simulink model "Linearisierung3_RoboKomplettmodell_Sim"  (R2017a)
settings: Solver=VariableStepAuto  StartTime=0.0  StopTime=50  RelTol=1e-3
values from neighbouring files (symbols this model uses):
  c = 1    [Linearisierung3_Robo.m]
  g = 9.81    [Linearisierung3_Robo.m]
  K = 300    [Linearisierung3_Robo.m]
  l = 1    [Linearisierung3_Robo.m]
  m = 7    [Linearisierung3_Robo.m]
  T = 0.1    [Linearisierung3_Robo.m]
settings Model: Creator=jonas  LastModifiedBy=Jonas

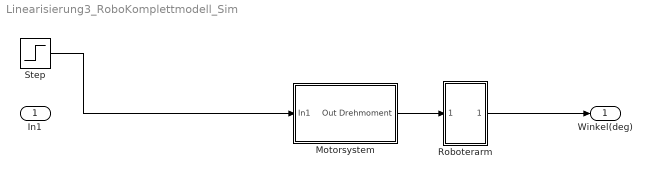
== system Linearisierung3_RoboKomplettmodell_Sim ==
  In1 : Inport
  Motorsystem : Subsystem
  Roboterarm : Subsystem
  Step : Step  After=0.1471  SampleTime=0
  Winkel(deg) : Outport
  wires:
  Motorsystem/1(Out Drehmoment) -> Roboterarm/1(In1)
  Roboterarm/1(Out1) -> Winkel(deg)/1
  Step/1 -> Motorsystem/1(In1)

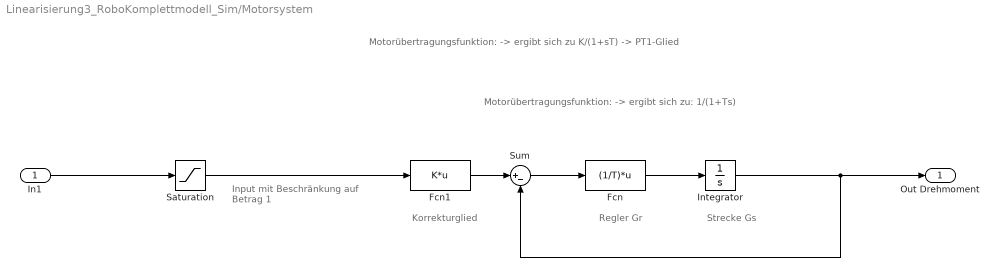
== system Linearisierung3_RoboKomplettmodell_Sim/Motorsystem ==
  note: Motorübertragungsfunktion:
      |  -> ergibt sich zu K/(1+sT)
      |  -> PT1-Glied
  note: Motorübertragungsfunktion:
      |  -> ergibt sich zu: 1/(1+Ts)
  note: Korrekturglied
  note: Input
      | mit Beschränkung
      | auf Betrag 1
  note: Regler Gr
  note: Strecke Gs
  In1 : Inport
  Fcn : Fcn  Expr=(1/T)*u
  Fcn1 : Fcn  Expr=K*u
  Integrator : Integrator
  Saturation : Saturate  UpperLimit=1  LowerLimit=-1
  Sum : Sum  Inputs=|+-
  Out Drehmoment : Outport
  wires:
  Fcn1/1 -> Sum/1
  Fcn/1 -> Integrator/1
  Integrator/1 -> Out Drehmoment/1, Sum/2
  Saturation/1 -> Fcn1/1
  Sum/1 -> Fcn/1
  In1/1 -> Saturation/1

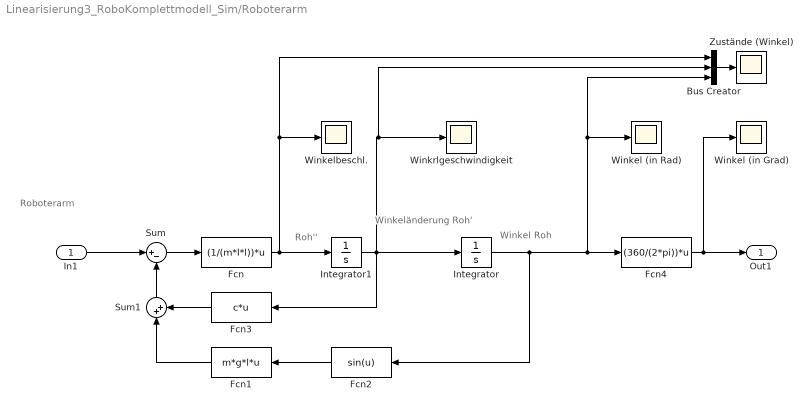
== system Linearisierung3_RoboKomplettmodell_Sim/Roboterarm ==
  note: Roboterarm
  note: Roh''
  note: Winkel Roh
  note: Winkeländerung
      | Roh'
  In1 : Inport
  Bus Creator : BusCreator  Inputs=3
  Fcn : Fcn  Expr=(1/(m*l*l))*u
  Fcn1 : Fcn  Expr=m*g*l*u
  Fcn2 : Fcn  Expr=sin(u)
  Fcn3 : Fcn  Expr=c*u
  Fcn4 : Fcn  Expr=(360/(2*pi))*u
  Integrator : Integrator
  Integrator1 : Integrator
  Sum : Sum  Inputs=|+-
  Sum1 : Sum  Inputs=|++
  Winkel (in Grad) : Scope
  "Winkel (in Rad) " : Scope
  Winkelbeschl. : Scope
  "Winkrlgeschwindigkeit " : Scope
  Zustände (Winkel) : Scope
  Out1 : Outport
  wires:
  Integrator/1 -> Fcn4/1, Bus Creator/3, "Winkel (in Rad) "/1, Fcn2/1
  Sum1/1 -> Sum/2
  Fcn1/1 -> Sum1/1
  Fcn3/1 -> Sum1/2
  Fcn2/1 -> Fcn1/1
  Sum/1 -> Fcn/1
  In1/1 -> Sum/1
  Fcn4/1 -> Winkel (in Grad)/1, Out1/1
  Integrator1/1 -> Bus Creator/2, "Winkrlgeschwindigkeit "/1, Fcn3/1, Integrator/1
  Fcn/1 -> Integrator1/1, Winkelbeschl./1, Bus Creator/1
  Bus Creator/1 -> Zustände (Winkel)/1
